simulink model "ex_4_sim"  (R2024b)
settings: Solver=ode23  StartTime=0.0  StopTime=20  RelTol=1e-3
values from neighbouring files (symbols this model uses):
  A = [0, 1 ... (first row only)    [Script.m]
  B = [0 ... (first row only)    [Script.m]
  C = [1, 0]    [Script.m]
  D = 0    [Script.m]
  den_filter = [1, 2*delta_filter*omega_filter, omega_filter^2]    [Script.m]
  denH = alpha    [Script.m]
  K_xi = K_z(m+1:end)    [Script.m]
  num_filter = [omega_filter^2, 0]    [Script.m]
undefined symbols (not defined in the file or in its folder): input_value, numH, step_amplitude
settings Model: Creator=andre  LastModifiedBy=andre

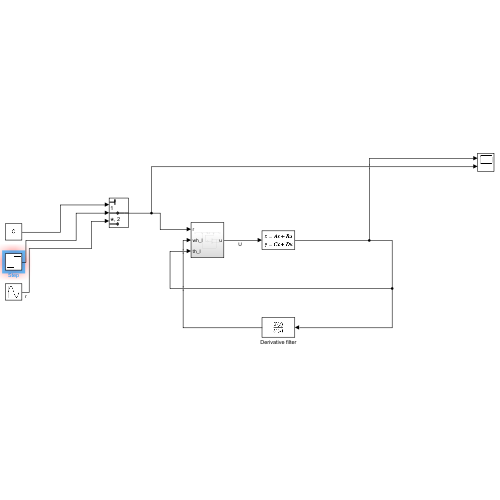
[thumbnail: Simulink's stored preview of the top-level diagram]
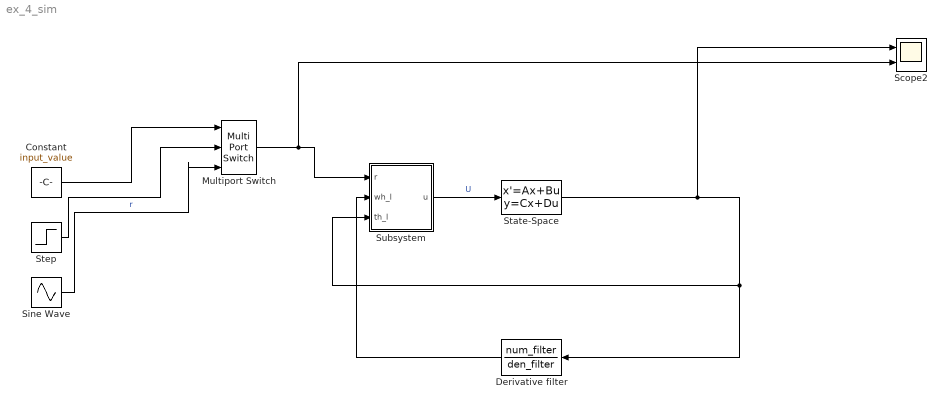
== system ex_4_sim ==
  Constant : Constant  Value=input_value
  Derivative filter : TransferFcn  Numerator=num_filter  Denominator=den_filter
  Multiport Switch : MultiPortSwitch  Inputs=2  SaturateOnIntegerOverflow=off  InputSameDT=off
  Scope2 : Scope  NumInputPorts=2
  Sine Wave : Sin  Amplitude=40  Frequency=6  SampleTime=0
  State-Space : StateSpace  A=A  B=B  C=C  D=D  InitialCondition=0
  Step : Step  Time=0  After=step_amplitude  SampleTime=0
  Subsystem : Subsystem
  wires:
  Subsystem/1(u) -> State-Space/1  "U"
  State-Space/1 -> Scope2/1, Subsystem/3(th_l), Derivative filter/1
  Derivative filter/1 -> Subsystem/2(wh_l)
  Constant/1 -> Multiport Switch/1
  Step/1 -> Multiport Switch/2
  Sine Wave/1 -> Multiport Switch/3  "r"
  Multiport Switch/1 -> Scope2/2, Subsystem/1(r)

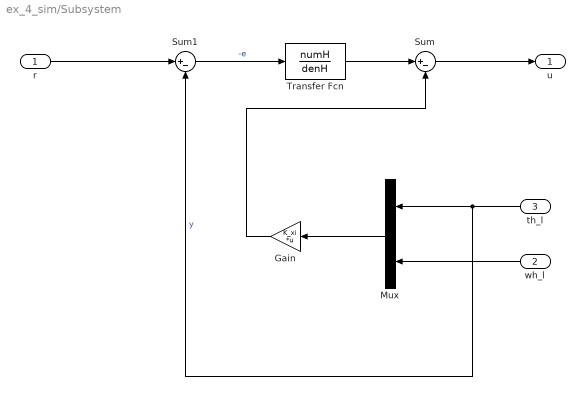
== system ex_4_sim/Subsystem ==
  r : Inport
  wh_l : Inport  Port=2
  th_l : Inport  Port=3
  Gain : Gain  Gain=K_xi  Multiplication=Matrix(K*u)
  Mux : Mux  Inputs=2
  Sum : Sum  Inputs=|+-
  Sum1 : Sum  Inputs=|+-
  Transfer Fcn : TransferFcn  Numerator=numH  Denominator=denH
  u : Outport
  wires:
  Gain/1 -> Sum/2
  Sum/1 -> u/1
  Mux/1 -> Gain/1
  Sum1/1 -> Transfer Fcn/1  "-e"
  wh_l/1 -> Mux/2
  Transfer Fcn/1 -> Sum/1
  r/1 -> Sum1/1
  th_l/1 -> Sum1/2, Mux/1  "y"
